simulink model "IMC_saturated_control101"  (R2024a)
settings: Solver=VariableStepAuto  StartTime=0.0  StopTime=endtime  RelTol=1e-3
undefined symbols (not defined in the file or in its folder): umax, umin
libraries: cstblocks x3
settings Model: Creator=barsr  LastModifiedBy=Anthony Rossiter
settings RTWCC: GPUComputeCapability=3.5

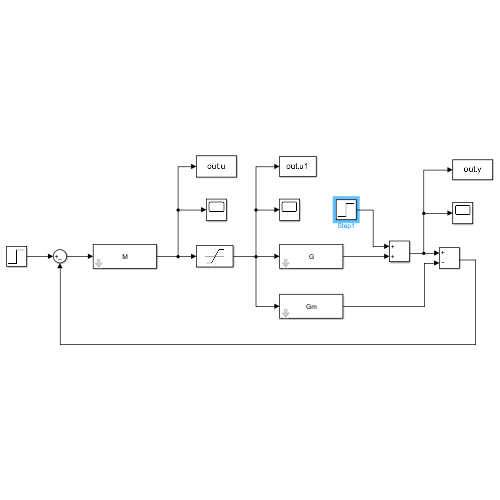
[thumbnail: Simulink's stored preview of the top-level diagram]
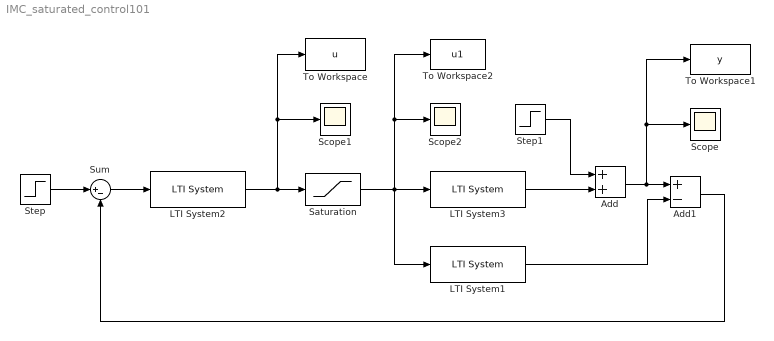
== system IMC_saturated_control101 ==
  Add : Sum
  Add1 : Sum  Inputs=+-
  LTI System1 : cstblocks/LTI System  sys=Gm  IC=[]  PadeOrder=0
  LTI System2 : cstblocks/LTI System  sys=M  IC=[]  PadeOrder=0
  LTI System3 : cstblocks/LTI System  sys=G  IC=[]  PadeOrder=0
  Saturation : Saturate  UpperLimit=umax  LowerLimit=umin
  Scope : Scope
  Scope1 : Scope
  Scope2 : Scope
  Step : Step  Time=0  SampleTime=0
  Step1 : Step  Time=10  After=0.5  SampleTime=0
  Sum : Sum  Inputs=|+-
  To Workspace : ToWorkspace  VariableName=u  SaveFormat=Structure With Time  SampleTime=-1
  To Workspace1 : ToWorkspace  VariableName=y  SaveFormat=Structure With Time  SampleTime=-1
  To Workspace2 : ToWorkspace  VariableName=u1  SaveFormat=Structure With Time  SampleTime=-1
  wires:
  Step/1 -> Sum/1
  Sum/1 -> LTI System2/1
  LTI System2/1 -> To Workspace/1, Scope1/1, Saturation/1
  Saturation/1 -> LTI System1/1, LTI System3/1, To Workspace2/1, Scope2/1
  LTI System3/1 -> Add/2
  Step1/1 -> Add/1
  Add/1 -> To Workspace1/1, Scope/1, Add1/1
  LTI System1/1 -> Add1/2
  Add1/1 -> Sum/2
